simulink model "Hierarchy4"  (Simulink 5.0)
settings: Solver=ode45  StartTime=0.0  StopTime=10.0  RelTol=1e-3
settings Model: Creator=scaife  LastModifiedBy=scaife  ExtModeAutoUpdateStatusClock=off

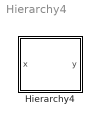
== system Hierarchy4 ==
  Hierarchy4 : Stateflow chart

== stateflow chart Hierarchy4 ==
  state A/
    en: y=1;
  state B/
    en: y=2;
  (default) -> A : [x==0]
  (default) -> B : [x<>0]
  data: x input int32; y output int32
